simulink model "CDCD_simulink (1)"  (R2024b)
settings: Solver=VariableStepAuto  StartTime=0.0  StopTime=0.01  RelTol=1e-3
InitFcn:
  | L = 0.002;
  | R = 10;
  | C = 0.000010;
  | Vin = 32;

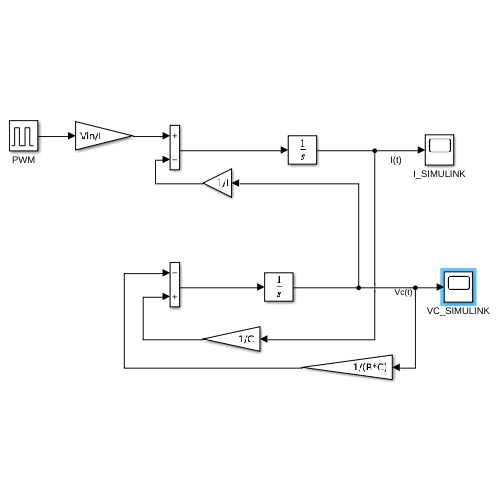
[thumbnail: Simulink's stored preview of the top-level diagram]
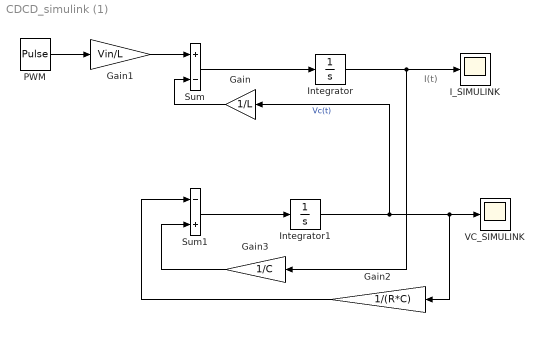
== system CDCD_simulink (1) ==
  note: I(t)
  Gain : Gain  Gain=1/L
  Gain1 : Gain  Gain=Vin/L
  Gain2 : Gain  Gain=1/(R*C)
  Gain3 : Gain  Gain=1/C
  I_SIMULINK : Scope
  Integrator : Integrator
  Integrator1 : Integrator
  PWM : DiscretePulseGenerator  PulseType=Time based  Amplitude=0.955  Period=1e-5  PulseWidth=50
  Sum : Sum  Inputs=+-
  Sum1 : Sum  Inputs=-+
  VC_SIMULINK : Scope
  wires:
  Gain1/1 -> Sum/1
  Gain/1 -> Sum/2
  Integrator/1 -> Gain3/1, I_SIMULINK/1
  PWM/1 -> Gain1/1
  Gain3/1 -> Sum1/2
  Sum/1 -> Integrator/1
  Integrator1/1 -> Gain2/1, VC_SIMULINK/1, Gain/1  "Vc(t)"
  Sum1/1 -> Integrator1/1
  Gain2/1 -> Sum1/1
